simulink model "simple_example_2"  (R2015a)
settings: Solver=ode45  StartTime=0.0  StopTime=120  RelTol=1e-3
InitFcn:
  | param
undefined symbols (not defined in the file or in its folder): ctrl, P
settings Model: Creator=beard  LastModifiedBy=beard
settings DebuggingCC: SignalLabelMismatchMsg=error

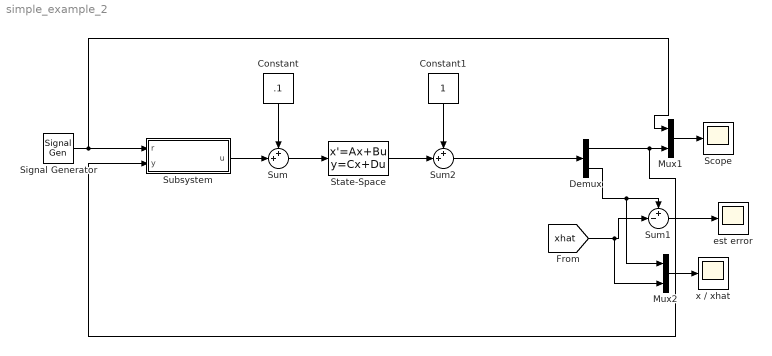
== system simple_example_2 ==
  Constant : Constant  Value=.1
  Constant1 : Constant
  Demux : Demux  Outputs=[1;2]
  Mux1 : Mux  Inputs=2
  Mux2 : Mux  Inputs=2
  Scope : Scope
      settings: TimeRange=120  YMin=-2  YMax=6
  Signal Generator : SignalGenerator  WaveForm=square  Frequency=.1  Units=rad/sec
  State-Space : StateSpace  A=P.A  B=P.B  C=[P.C; eye(2)]  D=[0;0;0]  X0=[0;0]
  Subsystem : Subsystem
  Sum : Sum  Inputs=++|
  Sum1 : Sum  Inputs=+-|
  Sum2 : Sum  Inputs=++|
  "est error " : Scope
      settings: TimeRange=120  YMin=-3  YMax=3
  x / xhat : Scope
      settings: TimeRange=120  YMin=-3  YMax=3  SaveName=ScopeData2
  wires:
  Signal Generator/1 -> Mux1/1, Subsystem/1(r)
  Mux1/1 -> Scope/1
  Demux/1 -> Subsystem/2(y), Mux1/2
  Demux/2 -> Mux2/1, Sum1/1
  Sum/1 -> State-Space/1
  Subsystem/1(u) -> Sum/2
  Sum1/1 -> "est error "/1
  [xhat] -> Mux2/2, Sum1/2
  Mux2/1 -> x / xhat/1
  Constant/1 -> Sum/1
  State-Space/1 -> Sum2/2
  Sum2/1 -> Demux/1
  Constant1/1 -> Sum2/1

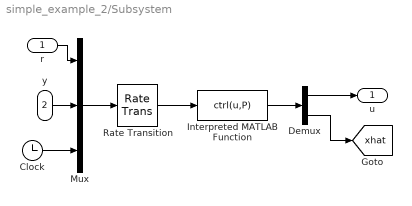
== system simple_example_2/Subsystem ==
  r : Inport
  y : Inport  Port=2
  Clock : Clock
  Demux : Demux  Outputs=[1;2]
  Interpreted MATLAB Function : MATLABFcn  MATLABFcn=ctrl(u,P)  OutputDimensions=1+2
  Mux : Mux  Inputs=3
  Rate Transition : RateTransition  OutPortSampleTime=P.Ts
  u : Outport
  tag scope: xhat=global
  wires:
  Rate Transition/1 -> Interpreted MATLAB Function/1
  r/1 -> Mux/1
  y/1 -> Mux/2
  Mux/1 -> Rate Transition/1
  Clock/1 -> Mux/3
  Interpreted MATLAB Function/1 -> Demux/1
  Demux/1 -> u/1
  Demux/2 -> [xhat]
